simulink model "chapter7_pitch_rate"  (R2021b)
settings: Solver=ode4  StartTime=0.0  StopTime=20  FixedStep=0.001  RelTol=1e-3
libraries: simulink x2
settings Model: Creator=cnsyk  LastModifiedBy=cnsyk

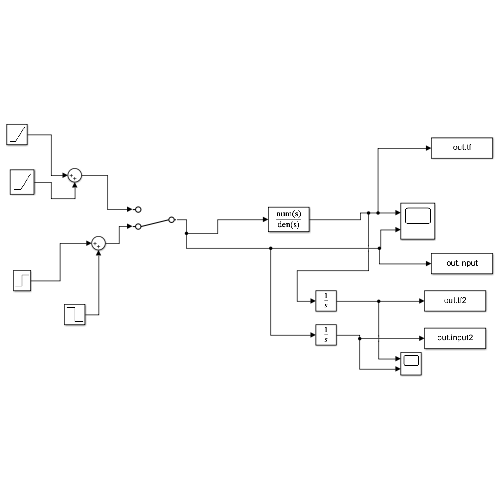
[thumbnail: Simulink's stored preview of the top-level diagram]
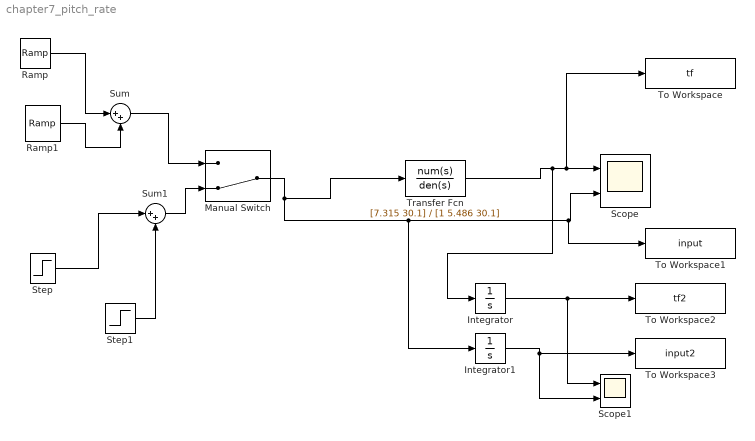
== system chapter7_pitch_rate ==
  Integrator : Integrator
  Integrator1 : Integrator
  Manual Switch : ManualSwitch  CurrentSetting=0
  Ramp : simulink/Sources/Ramp  slope=1  start=0  InitialOutput=0
  Ramp1 : simulink/Sources/Ramp  slope=-1  start=10  InitialOutput=0
  Scope : Scope  NumInputPorts=2
  Scope1 : Scope  NumInputPorts=2
  Step : Step  Time=0  SampleTime=0
  Step1 : Step  Time=5  After=-1  SampleTime=0
  Sum : Sum  Inputs=|++
  Sum1 : Sum  Inputs=|++
  To Workspace : ToWorkspace  VariableName=tf  SaveFormat=Timeseries  SampleTime=-1
  To Workspace1 : ToWorkspace  VariableName=input  SaveFormat=Timeseries  SampleTime=-1
  To Workspace2 : ToWorkspace  VariableName=tf2  SaveFormat=Timeseries  SampleTime=-1
  To Workspace3 : ToWorkspace  VariableName=input2  SaveFormat=Timeseries  SampleTime=-1
  Transfer Fcn : TransferFcn  Numerator=[7.315 30.1]  Denominator=[1 5.486 30.1]
  wires:
  Transfer Fcn/1 -> Integrator/1, To Workspace/1, Scope/1
  Ramp/1 -> Sum/1
  Ramp1/1 -> Sum/2
  Sum/1 -> Manual Switch/1
  Sum1/1 -> Manual Switch/2
  Step/1 -> Sum1/1
  Step1/1 -> Sum1/2
  Manual Switch/1 -> Transfer Fcn/1, Integrator1/1, To Workspace1/1, Scope/2
  Integrator/1 -> Scope1/1, To Workspace2/1
  Integrator1/1 -> Scope1/2, To Workspace3/1
